simulink library "storePerformanceIndex"  (R2018a)
settings: Solver=VariableStepAuto  StartTime=0.0  StopTime=10.0  RelTol=1e-3
settings Model: Creator=mitch  LastModifiedBy=mitch

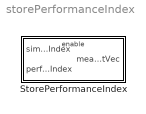
== system storePerformanceIndex ==
  StorePerformanceIndex : Subsystem

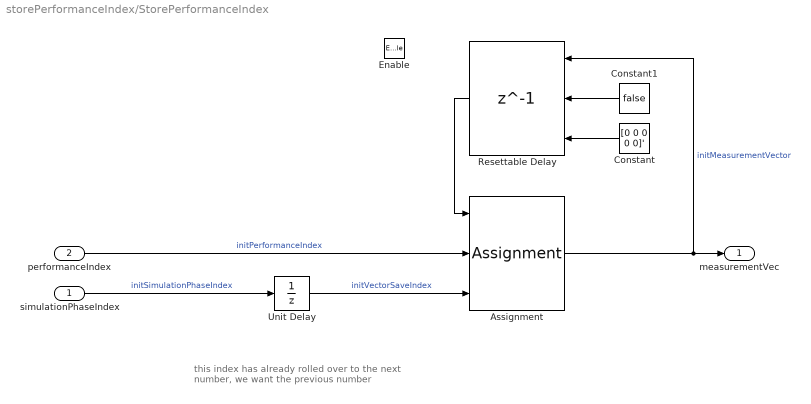
== system storePerformanceIndex/StorePerformanceIndex ==
  note: this index has already rolled over to the
      | next number, we want the previous number
  simulationPhaseIndex : Inport
  performanceIndex : Inport  Port=2
  Enable : EnablePort
  Assignment : Assignment  DiagnosticForDimensions=Warning  IndexOptions=Index vector (port)  Indices=1  OutputSizes=1
  Constant : Constant  Value=[0 0 0 0 0]'
  Constant1 : Constant  Value=false
  Resettable Delay : Delay  DelayLength=1  InitialConditionSource=Input port  ExternalReset=Rising
      settings: InputPortMap=u0,r5,p4
  Unit Delay : UnitDelay  InitialCondition=1  SampleTime=-1
  measurementVec : Outport
  wires:
  simulationPhaseIndex/1 -> Unit Delay/1  "initSimulationPhaseIndex"
  performanceIndex/1 -> Assignment/2  "initPerformanceIndex"
  Unit Delay/1 -> Assignment/3  "initVectorSaveIndex"
  Assignment/1 -> Resettable Delay/1, measurementVec/1  "initMeasurementVector"
  Resettable Delay/1 -> Assignment/1
  Constant/1 -> Resettable Delay/3
  Constant1/1 -> Resettable Delay/2
